simulink model "Conexion_Unity"  (R2020b)
settings: Solver=VariableStepAuto  StartTime=0.0  StopTime=10.0  RelTol=1e-3
libraries: etargetslib x1, dspnetwork x1
settings Model: EnablePacing=on  Creator=jaime  LastModifiedBy=jaime

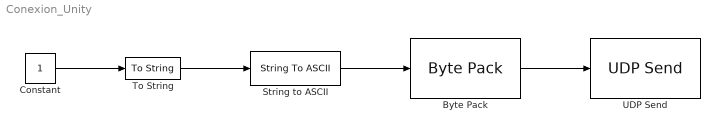
== system Conexion_Unity ==
  Byte Pack : etargetslib/Byte Pack  datatypes={'uint8'}  byteAlign=1
  Constant : Constant
  String to ASCII : StringToASCII  OutputVectorSize=64
  To String : ToString
  UDP Send : dspnetwork/UDP Send  remoteURL='127.0.0.1'  remotePort=1234  localURL='0.0.0.0'  localPortSource=Automatically determine  localPort=-1  sendBufferSize=8192  sampletime=-1  blockPlatform=HOST  separateLengthPort=0
  wires:
  Constant/1 -> To String/1
  To String/1 -> String to ASCII/1
  String to ASCII/1 -> Byte Pack/1
  Byte Pack/1 -> UDP Send/1
